simulink model "p4p3"  (R2014a)
settings: Solver=ode1  StartTime=0.0  StopTime=inf  FixedStep=0.002  RelTol=1e-3
PostLoadFcn:
  | qc_set_target_type(getConfigSet(bdroot, 'QUARC Default Target Configuration'));
undefined symbols (not defined in the file or in its folder): A4_2, B4_2, C4_3, HIL, Joystick_gain_x, Joystick_gain_y, K3_3, L4_3, P3_3, qc_get_step_size, Vs_star
libraries: simulink_extras x6, quarc_library x4
settings Model: SimulationMode=external  ExtModeTrigDuration=5000  Creator=Rchan  LastModifiedBy=arefv
settings SolverCC: PositivePriorityOrder=on
settings DataIOCC: MaxDataPoints=3000  SignalLoggingSaveFormat=ModelDataLogs
settings OptimizationCC: ExpressionDepthLimit=2147483647  InitFltsAndDblsToZero=on
settings DebuggingCC: SaveWithParameterizedLinksMsg=none  UnderspecifiedInitializationDetection=Classic  MultiTaskDSMMsg=warning  MultiTaskCondExecSysMsg=none  FcnCallInpInsideContextMsg=UseLocalSettings  StateNameClashWarn=warning
settings RTWCC: SystemTargetFile=quarc_win64.tlc  TemplateMakefile=quarc_default_tmf  Description=QUARC Win64 Target  ProcessScript=quarc_win64_make_rtw_hook
settings STFCustomTargetCC: CPPClassGenCompliant=on
settings GRTTargetCC: ParMdlRefBuildCompliant=off  CompOptLevelCompliant=off  CombineOutputUpdateFcns=off  MatFileLogging=off  GRTInterface=on  ExtMode=on  ExtModeMexFile=quarc_comm

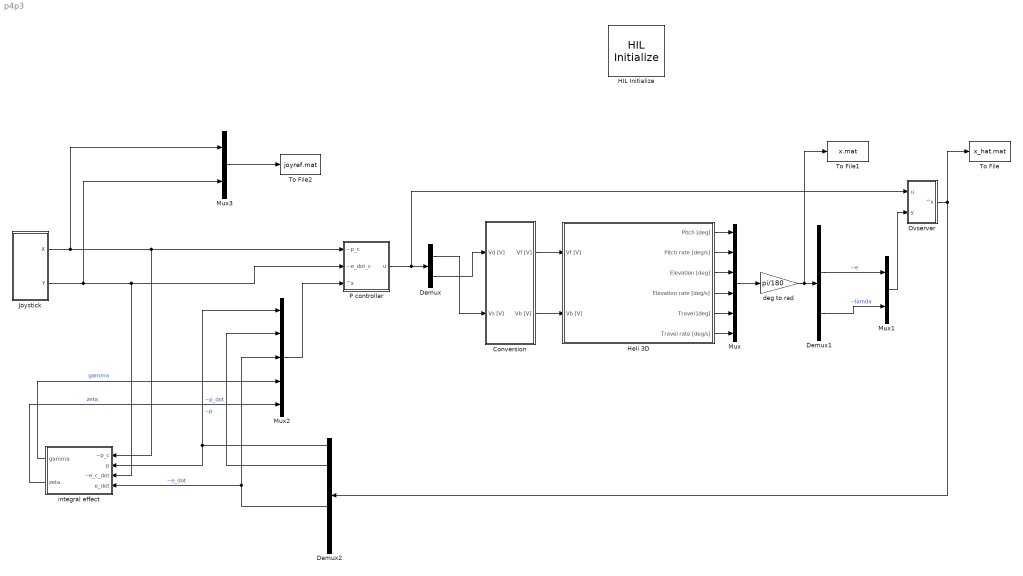
== system p4p3 ==
  Conversion : Subsystem
  Demux : Demux  Outputs=2
  Demux1 : Demux  Outputs=6
  Demux2 : Demux  Outputs=6
  HIL Initialize : quarc_library/Data Acquisition/Generic/Configuration/HIL Initialize  Priority=-99  object_name=HIL-1  board_type=q8_usb  board_number=0  board_options=update_rate=normal;decimation=1  exclusive=off  active=off  hardware_clocks=[0:2]  clock_modes=[]  initial_clock_frequencies=[]  set_clock_params_at_start=off  set_clock_params_at_switch_in=off  set_clock_frequencies_at_start=off  set_clock_frequencies_at_switch_in=off  analog_input_channels=[0:7]  analog_input_maximums=10  analog_input_minimums=-10  set_analog_input_params_at_start=on  set_analog_input_params_at_switch_in=off  analog_output_channels=[0:7]  analog_output_maximums=10  analog_output_minimums=-10  initial_analog_outputs=[0]  final_analog_outputs=[0]  watchdog_analog_outputs=0  set_analog_output_params_at_start=on  set_analog_output_params_at_switch_in=off  set_analog_outputs_at_start=on  set_analog_outputs_at_switch_in=off  set_analog_outputs_at_terminate=on  set_analog_outputs_at_switch_out=off  set_analog_outputs_on_watchdog=off  digital_input_channels=[]  digital_output_channels=[]  digital_output_configuration=[]  initial_digital_outputs=[1]  final_digital_outputs=[1]  watchdog_digital_outputs=[1]  set_digital_output_params_at_start=off  set_digital_output_params_at_switch_in=off  set_digital_outputs_at_start=on  set_digital_outputs_at_switch_in=off  set_digital_outputs_at_terminate=on  set_digital_outputs_at_switch_out=off  set_digital_outputs_on_watchdog=off  encoder_channels=[0:7]  quadrature=[4]  encoder_filter_frequency=[]  initial_encoder_counts=[0]  set_encoder_params_at_start=on  set_encoder_params_at_switch_in=off  set_encoder_counts_at_start=on  set_encoder_counts_at_switch_in=off  pwm_channels=[0:7]  pwm_modes=0  pwm_frequency=99.532799999999995e6/4095  pwm_configuration=[0]  pwm_alignment=[0]  pwm_polarity=[1]  pwm_leading_deadband=[0]  pwm_trailing_deadband=[0]  initial_pwm_outputs=[0]  final_pwm_outputs=[0]  watchdog_pwm_outputs=[0]  set_pwm_params_at_start=on  set_pwm_params_at_switch_in=off  set_pwm_outputs_at_start=on  set_pwm_outputs_at_switch_in=off  set_pwm_outputs_at_terminate=on  set_pwm_outputs_at_switch_out=off  set_pwm_outputs_on_watchdog=off  other_output_channels=[]  initial_other_outputs=[]  final_other_outputs=[]  watchdog_other_outputs=[]  set_other_outputs_at_start=off  set_other_outputs_at_switch_in=off  set_other_outputs_at_terminate=off  set_other_outputs_at_switch_out=off  set_other_outputs_on_watchdog=off
  Heli 3D : Subsystem
  Joystick : Subsystem
  Mux : Mux  Inputs=6
  Mux1 : Mux  Inputs=2
  Mux2 : Mux  Inputs=5
  Mux3 : Mux  Inputs=2
  Ovserver : Subsystem
  P controller : Subsystem
  To File : ToFile  Filename=x_hat.mat  MatrixName=x_h
  To File1 : ToFile  Filename=x.mat  MatrixName=x
  To File2 : ToFile  Filename=joyref.mat  MatrixName=joyref
  deg to rad : Gain  Gain=pi/180
  integral effect : Subsystem
  wires:
  Conversion/2(Vb [V]) -> Heli 3D/2(Vb [V])
  Conversion/1(Vf [V]) -> Heli 3D/1(Vf [V])
  Mux/1 -> deg to rad/1
  Demux/1 -> Conversion/2(Vs [V])
  Demux/2 -> Conversion/1(Vd [V])
  Joystick/1(X) -> Mux3/1, P controller/1(~p_c), integral effect/1(~p_c)
  Joystick/2(Y) -> integral effect/3(~e_c_dot), P controller/2(~e_dot_c), Mux3/2
  deg to rad/1 -> To File1/1, Demux1/1
  Mux1/1 -> Ovserver/2(y)
  P controller/1(u) -> Ovserver/1(u), Demux/1
  Ovserver/1(^x) -> To File/1, Demux2/1
  Demux2/1 -> Mux2/1, integral effect/2(p)  "~p"
  Demux2/4 -> integral effect/4(e_dot), Mux2/3  "~e_dot"
  Demux2/2 -> Mux2/2  "~p_dot"
  integral effect/1(gamma) -> Mux2/4  "gamma"
  integral effect/2(zeta) -> Mux2/5  "zeta"
  Mux2/1 -> P controller/3(^x)
  Heli 3D/6(Travel rate [deg/s]) -> Mux/6
  Heli 3D/5(Travel [deg]) -> Mux/5
  Heli 3D/4(Elevation rate [deg/s]) -> Mux/4
  Heli 3D/3(Elevation [deg]) -> Mux/3
  Heli 3D/2(Pitch rate [deg/s]) -> Mux/2
  Heli 3D/1(Pitch [deg]) -> Mux/1
  Demux1/5 -> Mux1/2  "~lamda"
  Mux3/1 -> To File2/1
  Demux1/3 -> Mux1/1  "~e"

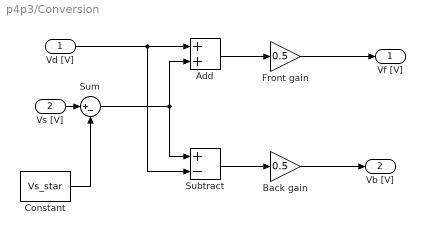
== system p4p3/Conversion ==
  Vd [V] : Inport
  Vs [V] : Inport  Port=2
  Add : Sum
  Back gain : Gain  Gain=0.5
  Constant : Constant  Value=Vs_star
  Front gain : Gain  Gain=0.5
  Subtract : Sum  Inputs=+-
  Sum : Sum  Inputs=|+-
  Vf [V] : Outport
  Vb [V] : Outport  Port=2
  wires:
  Vd [V]/1 -> Subtract/2, Add/1
  Subtract/1 -> Back gain/1
  Back gain/1 -> Vb [V]/1
  Add/1 -> Front gain/1
  Front gain/1 -> Vf [V]/1
  Vs [V]/1 -> Sum/1
  Constant/1 -> Sum/2
  Sum/1 -> Add/2, Subtract/1

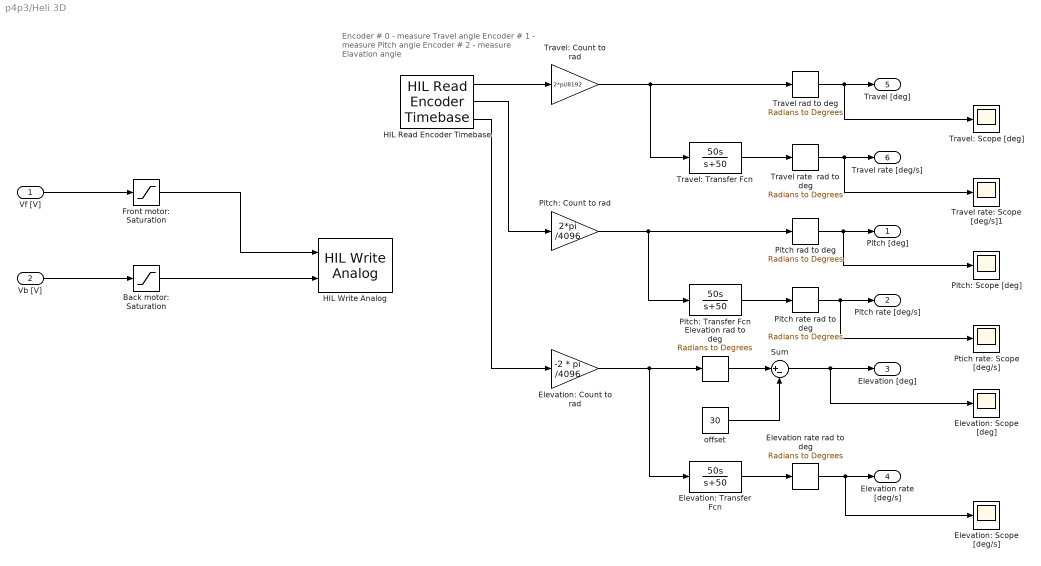
== system p4p3/Heli 3D ==
  note: Encoder # 0 - measure Travel angle
      | Encoder # 1 - measure Pitch angle
      | Encoder # 2 - measure Elavation angle
  Vf [V] : Inport
  Vb [V] : Inport  Port=2
  Back motor: Saturation : Saturate  UpperLimit=5  LowerLimit=-5
  Elevation rad to deg : simulink_extras/Transformations/Radians to Degrees
  Elevation rate rad to deg : simulink_extras/Transformations/Radians to Degrees
  Elevation: Count to rad : Gain  Gain=-2 * pi /4096
  Elevation: Scope [deg/s] : Scope
      settings: YMin=-15  YMax=15  SaveName=ScopeData13
  Elevation: Scope [deg] : Scope
      settings: YMin=-15  YMax=15  SaveName=ScopeData12
  Elevation: Transfer Fcn : TransferFcn  Numerator=[50 0]  Denominator=[1 50]
  Front motor: Saturation : Saturate  UpperLimit=5  LowerLimit=-5
  HIL Read Encoder Timebase : quarc_library/Data Acquisition/Generic/Timebases/HIL Read Encoder Timebase  object_name=HIL-1  clock=0  channels=[0:2]  samples_in_buffer=max(ceil(1/qc_get_step_size), 1)  active=on  vector_output=off  data_type_mode=Inherit via back propagation  data_type=double
  HIL Write Analog : quarc_library/Data Acquisition/Generic/Immediate I//O/HIL Write Analog  object_name=HIL-1  channels=[0:1]  sample_time=-1  active=off  vector_input=off
  Pitch rad to deg : simulink_extras/Transformations/Radians to Degrees
  Pitch rate rad to deg : simulink_extras/Transformations/Radians to Degrees
  Pitch: Count to rad : Gain  Gain=2*pi /4096
  Pitch: Scope [deg] : Scope
      settings: YMin=-15  YMax=15  SaveName=ScopeData10
  Pitch: Transfer Fcn : TransferFcn  Numerator=[50 0]  Denominator=[1 50]
  Ptich rate: Scope [deg/s] : Scope
      settings: YMin=-15  YMax=15  SaveName=ScopeData11
  Sum : Sum  Inputs=|+-
  Travel rad to deg : simulink_extras/Transformations/Radians to Degrees
  Travel rate  rad to deg : simulink_extras/Transformations/Radians to Degrees
  Travel rate: Scope [deg/s]1 : Scope
      settings: YMin=-15  YMax=15  SaveName=ScopeData3
  Travel: Count to rad : Gain  Gain=2*pi/8192
  Travel: Scope [deg] : Scope
      settings: YMin=-15  YMax=15  SaveName=ScopeData8
  Travel: Transfer Fcn : TransferFcn  Numerator=[50 0]  Denominator=[1 50]
  offset : Constant  Value=30
  Pitch [deg] : Outport
  Pitch rate [deg/s] : Outport  Port=2
  Elevation [deg] : Outport  Port=3
  Elevation rate [deg/s] : Outport  Port=4
  Travel [deg] : Outport  Port=5
  Travel rate [deg/s] : Outport  Port=6
  wires:
  HIL Read Encoder Timebase/1 -> Travel: Count to rad/1
  HIL Read Encoder Timebase/2 -> Pitch: Count to rad/1
  HIL Read Encoder Timebase/3 -> Elevation: Count to rad/1
  Travel: Count to rad/1 -> Travel: Transfer Fcn/1, Travel rad to deg/1
  Travel: Transfer Fcn/1 -> Travel rate  rad to deg/1
  Pitch: Count to rad/1 -> Pitch: Transfer Fcn/1, Pitch rad to deg/1
  Pitch: Transfer Fcn/1 -> Pitch rate rad to deg/1
  Elevation: Count to rad/1 -> Elevation: Transfer Fcn/1, Elevation rad to deg/1
  Elevation: Transfer Fcn/1 -> Elevation rate rad to deg/1
  Travel rad to deg/1 -> Travel: Scope [deg]/1, Travel [deg]/1
  Travel rate  rad to deg/1 -> Travel rate: Scope [deg/s]1/1, Travel rate [deg/s]/1
  Pitch rad to deg/1 -> Pitch: Scope [deg]/1, Pitch [deg]/1
  Pitch rate rad to deg/1 -> Ptich rate: Scope [deg/s]/1, Pitch rate [deg/s]/1
  Elevation rate rad to deg/1 -> Elevation: Scope [deg/s]/1, Elevation rate [deg/s]/1
  Vf [V]/1 -> Front motor: Saturation/1
  Vb [V]/1 -> Back motor: Saturation/1
  Front motor: Saturation/1 -> HIL Write Analog/1
  Back motor: Saturation/1 -> HIL Write Analog/2
  offset/1 -> Sum/2
  Elevation rad to deg/1 -> Sum/1
  Sum/1 -> Elevation: Scope [deg]/1, Elevation [deg]/1

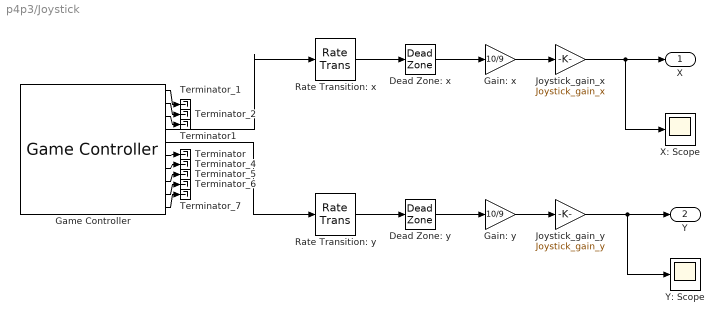
== system p4p3/Joystick ==
  Dead Zone: x : DeadZone  LowerValue=-0.1  UpperValue=0.1  SaturateOnIntegerOverflow=on
  Dead Zone: y : DeadZone  LowerValue=-0.1  UpperValue=0.1  SaturateOnIntegerOverflow=on
  Gain: x : Gain  Gain=10/9
  Gain: y : Gain  Gain=10/9
  Game Controller : quarc_library/Devices/Peripherals/Target/Game Controller  controller=1  buffer_size=12  deadzone=[]  saturation=[]  sample_time=max(qc_get_step_size, 0.01)  auto_center=off  enabled=on
  Joystick_gain_x : Gain  Gain=Joystick_gain_x
  Joystick_gain_y : Gain  Gain=Joystick_gain_y
  Rate Transition: x : RateTransition
  Rate Transition: y : RateTransition
  Terminator : Terminator
  Terminator1 : Terminator
  Terminator_{1..2,4..7} (6 alike) : Terminator
  X: Scope : Scope
      settings: YMin=-1  YMax=1  SaveName=ScopeData7
  Y: Scope : Scope
      settings: YMin=-10  YMax=10  SaveName=ScopeData5
  X : Outport
  Y : Outport  Port=2
  wires:
  Rate Transition: y/1 -> Dead Zone: y/1
  Rate Transition: x/1 -> Dead Zone: x/1
  Game Controller/5 -> Rate Transition: y/1
  Game Controller/4 -> Rate Transition: x/1
  Game Controller/1 -> Terminator_1/1
  Game Controller/2 -> Terminator_2/1
  Game Controller/7 -> Terminator_4/1
  Game Controller/8 -> Terminator_5/1
  Game Controller/9 -> Terminator_6/1
  Game Controller/10 -> Terminator_7/1
  Game Controller/3 -> Terminator1/1
  Game Controller/6 -> Terminator/1
  Dead Zone: x/1 -> Gain: x/1
  Dead Zone: y/1 -> Gain: y/1
  Gain: x/1 -> Joystick_gain_x/1
  Gain: y/1 -> Joystick_gain_y/1
  Joystick_gain_x/1 -> X/1, X: Scope/1
  Joystick_gain_y/1 -> Y: Scope/1, Y/1

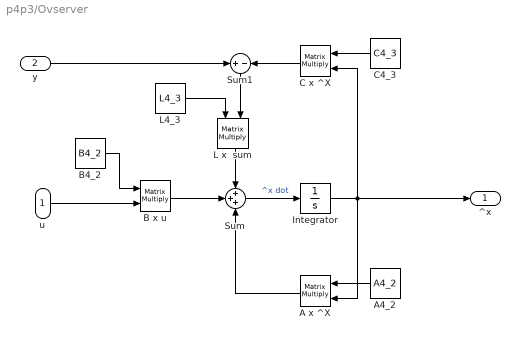
== system p4p3/Ovserver ==
  u : Inport
  y : Inport  Port=2
  A x ^X : Product  Multiplication=Matrix(*)
  A4_2 : Constant  Value=A4_2
  B x u : Product  Multiplication=Matrix(*)
  B4_2 : Constant  Value=B4_2
  C x ^X : Product  Multiplication=Matrix(*)
  C4_3 : Constant  Value=C4_3
  Integrator : Integrator
  L x  sum : Product  Multiplication=Matrix(*)
  L4_3 : Constant  Value=L4_3
  Sum : Sum  Inputs=+++
  Sum1 : Sum  Inputs=+|-
  ^x : Outport
  wires:
  A x ^X/1 -> Sum/3
  C x ^X/1 -> Sum1/2
  Sum/1 -> Integrator/1  "^x dot"
  Integrator/1 -> ^x/1, A x ^X/2, C x ^X/2
  u/1 -> B x u/2
  L x  sum/1 -> Sum/1
  A4_2/1 -> A x ^X/1
  C4_3/1 -> C x ^X/1
  B x u/1 -> Sum/2
  B4_2/1 -> B x u/1
  y/1 -> Sum1/1
  Sum1/1 -> L x  sum/2
  L4_3/1 -> L x  sum/1

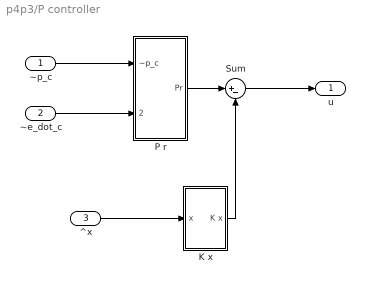
== system p4p3/P controller ==
  ~p_c : Inport
  ~e_dot_c : Inport  Port=2
  ^x : Inport  Port=3
  K x : Subsystem
  P r : Subsystem
  Sum : Sum  Inputs=|+-
  u : Outport
  wires:
  ~e_dot_c/1 -> P r/2(~e_dot_c)
  ~p_c/1 -> P r/1(~p_c)
  Sum/1 -> u/1
  P r/1(Pr) -> Sum/1
  K x/1(K x) -> Sum/2
  ^x/1 -> K x/1(x)

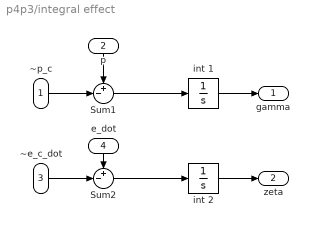
== system p4p3/integral effect ==
  ~p_c : Inport
  p : Inport  Port=2
  ~e_c_dot : Inport  Port=3
  e_dot : Inport  Port=4
  Sum1 : Sum  Inputs=+-|
  Sum2 : Sum  Inputs=+-|
  int 1 : Integrator
  int 2 : Integrator
  gamma : Outport
  zeta : Outport  Port=2
  wires:
  Sum2/1 -> int 2/1
  p/1 -> Sum1/1
  ~e_c_dot/1 -> Sum2/2
  e_dot/1 -> Sum2/1
  ~p_c/1 -> Sum1/2
  int 2/1 -> zeta/1
  int 1/1 -> gamma/1
  Sum1/1 -> int 1/1

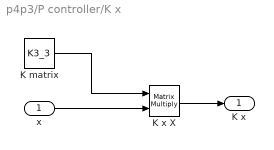
== system p4p3/P controller/K x ==
  x : Inport
  K matrix : Constant  Value=K3_3
  K x X : Product  Multiplication=Matrix(*)
  K x : Outport
  wires:
  K matrix/1 -> K x X/1
  x/1 -> K x X/2
  K x X/1 -> K x/1

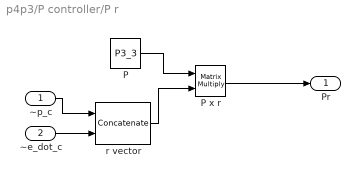
== system p4p3/P controller/P r ==
  ~p_c : Inport
  ~e_dot_c : Inport  Port=2
  P : Constant  Value=P3_3
  P x r : Product  Multiplication=Matrix(*)
  r vector : Concatenate  ConcatenateDimension=2
  Pr : Outport
  wires:
  ~p_c/1 -> r vector/1
  ~e_dot_c/1 -> r vector/2
  P x r/1 -> Pr/1
  P/1 -> P x r/1
  r vector/1 -> P x r/2
